simulink library "BaseOperationLib_Browser"  (Simulink 7.5)
settings: Solver=ode45  StartTime=0.0  StopTime=10.0  RelTol=1e-3
undefined symbols (not defined in the file or in its folder): DiscIntNeverNeededParam
libraries: BaseOperationLib_Browser x6, simulink x2
settings Model: Creator=zhangliming  LastModifiedBy=xinming

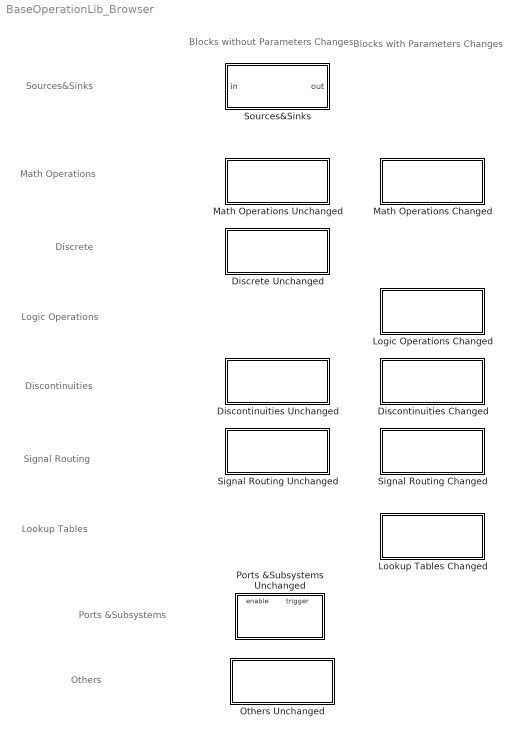
== system BaseOperationLib_Browser ==
  note: Sources&Sinks
  note: Math Operations
  note: Discrete
  note: Discontinuities
  note: Signal Routing
  note: Lookup Tables
  note: Others
  note: Ports &Subsystems
  note: Blocks without
      | Parameters Changes
  note: Blocks with
      | Parameters Changes
  note: Logic Operations
  Discontinuities Changed : Subsystem
  Discontinuities Unchanged : Subsystem
  "Discrete Unchanged " : Subsystem
  Logic Operations Changed : Subsystem
  Lookup Tables Changed : Subsystem
  Math Operations Changed : Subsystem
  Math Operations Unchanged : Subsystem
  Others Unchanged : Subsystem
  Ports &Subsystems Unchanged : Subsystem  TreatAsAtomicUnit=on
  Signal Routing Changed : Subsystem
  Signal Routing Unchanged : Subsystem
  Sources&Sinks : Subsystem

== system BaseOperationLib_Browser/Discontinuities Changed ==
  Relay : Relay  OnSwitchValue=1  OffSwitchValue=1  OutDataType=fixdt(1, 16)  OutScaling=2^0  OutDataTypeStr=Inherit: Inherit via back propagation
      settings: AttributesFormatString=%<OnSwitchValue> OnOut %<OnOutputValue>\n%<OffSwitchValue> OffOut %<OffOutputValue>
      mask Display: patch([0 1 1 1 .75], [1 1 0 .75 1], [0 1 0]);

== system BaseOperationLib_Browser/Discontinuities Unchanged ==
  RampLim : Subsystem
  Rate Limiter Dynamic : Subsystem
      mask Type: Rate Limiter Dynamic
      mask Description: Limit rising and falling rates of the signals at the second input by using the first input (upper limit) and the third input (lower limit).
      mask Display:
      | patch([0 1 1 1 .75], [1 1 0 .75 1], [0 1 0]);
      | plot([0.15 0.95],[.5 .5],[.5 .5],[0.05 0.95],0.05+0.9*[.2 .8],0.05+0.9*[0 1]);
  Saturation : Saturate  OutDataType=fixdt(1, 16)  OutScaling=2^0
      settings: AttributesFormatString=ULim:%<UpperLimit>\nLLim:%<LowerLimit>
      mask Display: patch([0 1 1 1 .75], [1 1 0 .75 1], [0 1 0]);
  Saturation Dynamic : Subsystem  mask(Saturation Dynamic){OutMin=[], OutMax=[], OutDataTypeStr=Inherit: Same as second input, OutputDataTypeScalingMode=Same as second input, OutDataType=fixdt(1, 16), OutScaling=2^-10, LockScale=off, RndMeth=Floor, DoSatur=on}
      mask prompts: OutMin "Output minimum:"; OutMax "Output maximum:"; OutDataTypeStr "Output data type:"; OutputDataTypeScalingMode "Output data type mode:"; OutDataType "Output data type (e.g. fixdt(1, 16), fixdt('single')):"; OutScaling "Output scaling (Slope, e.g. 2^-9 or [Slope Bias], e.g. [1.25 3]):"; LockScale "Lock output data type setting against changes by the fixed-point tools"; RndMeth "Integer rounding mode:"; DoSatur "Saturate on integer overflow"
      mask help: Bound the range of the second input by using the first input (upper limit) and the third input (lower limit).
      mask init:
      | blkH = gcbh;
      | blkName = getfullname(blkH);
      | 
      | switch_blks = {'Switch','Switch2'}; 
      | for i = 1:length(switch_blks)
      |   set_param([blkName,'/',switch_blks{i}], ...
      |       'RndMeth', RndMeth, ...
      | 	  'DoSatur', DoSatur);
      | end
      | 
      | propBlk = [blkName, '/Data Type Propagation'];
      | 
      | if strcmp(OutputDataTypeScalingMode, 'Same as second input')
      |     set_param(propBlk, 'PropDataTypeMode', 'Inherit via propagation rule', ...
      |                        'PropScalingMode',  'Inherit via propagation rule');
      | else
      |     scaling = OutScaling;
      |     switch OutputDataTypeScalingMode
      |       case 'double'
      |         dataType = 'fixdt(''double'')';
      |       case 'single'
      |         dataType = 'fixdt(''single'')';
      |       case 'int8'
      |         dataType = 'fixdt(1,8,0)';
      |       case 'uint8'
      |         dataType = 'fixdt(0,8,0)';
      |       case 'int16'
      |         dataType = 'fixdt(1,16,0)';
      |       case 'uint16'
      |         dataType = 'fixdt(0,16,0)';
      |       case 'int32'
      |         dataType = 'fixdt(1,32,0)';
      |       case 'uint32'
      |         dataType = 'fixdt(0,32,0)';
      |       case 'Specify via dialog'
      |         dataType = OutDataType;
      |     end
      |     
      |     set_param(propBlk, 'PropDataTypeMode', 'Specify via dialog', ...
      |                        'PropScalingMode',  'Specify via dialog', ...
      |                        'PropDataType',     dataType, ...
      |                        'PropScaling',      scaling);
      | end
      mask StyleString: min,max,unidt({m=3|4|5||6|1|2|}{i=Inherit: Same as second input}{b=double|single|int8|uint8|int16|uint16|int32|uint32}{s=UDTBinaryPointMode|UDTSlopeBiasMode}{g=UDTSignedSign|UDTUnsignedSign}),popup(double|single|int8|uint8|int16|uint16|int32|uint32|Specify via dialog|Same as second input),edit,edit,checkbox,popup(Ceiling|Convergent|Floor|Nearest|Round|Simplest|Zero),checkbox
      mask CallbackString: ||fixptdialog(gcbh)|fixptdialog(gcbh)|fixptdialog(gcbh)||||
      mask TabNameString: Signal Attributes,Signal Attributes,Signal Attributes,Signal Attributes,Signal Attributes,Signal Attributes,Signal Attributes,Signal Attributes,Signal Attributes
      mask Display:
      | patch([0 1 1 1 .75], [1 1 0 .75 1], [0 1 0]);
      | plot([0.15 0.85],[.5 .5],[.5 .5],[0.05 0.95],0.15+0.7*[0 .25 .75 1],0.05+0.9*[.25 .25 .75 .75]);
  WerghtingFilter : Subsystem

== system BaseOperationLib_Browser/Discrete Unchanged  ==
  note: Nothing else, only "limit out" could not be chose. It can be limit outside this block.
  Discrete-Time Integrator1 : DiscreteIntegrator  ExternalReset=falling  SampleTime=-1  OutDataType=PDT_s  OutDataTypeStr=Inherit: Inherit via back propagation  UpperSaturationLimit=100  LowerSaturationLimit=0  ICPrevOutput=DiscIntNeverNeededParam  ICPrevScaledInput=DiscIntNeverNeededParam
  Unit Delay : UnitDelay  SampleTime=-1
      mask Display: patch([0 1 1 1 .75], [1 1 0 .75 1], [0 1 0]);
  Unit Delay External IC : Subsystem  mask(Unit Delay External Initial Condition){tsamp=-1}
      mask prompts: tsamp "Sample time:"
      mask help:
      | Normally, the output is the signal u delayed by one sample period.
      | The initial condition is given by the signal IC.
      mask Display:
      | patch([0 1 1 1 .75], [1 1 0 .75 1], [0 1 0]);
      | dpoly(1,[1 0],'z')

== system BaseOperationLib_Browser/Logic Operations Changed ==
  Compare To Constant : Subsystem  mask(Compare To Constant){relop=<=, const=3.0, ZeroCross=on}
      mask prompts: relop "Operator:"; const "Constant value:"; ZeroCross "Enable zero-crossing detection"
      mask help: Determine how a signal compares to a constant.
      mask init:
      | blkName = gcb;
      | 
      | set_param([blkName,'/Compare'],'relop',relop, ...
      | 	 'ZeroCross', ZeroCross);
      | 
      | str = [relop,' C']; %default
      | 
      | const_str = get_param(blkName, 'const');
      | 
      | if isempty(strfind(const_str, ' ')) && isempty(strfind(const_str, ','))
      |     % scalar or single expression
      |     if isempty(str2num(const_str))
      |         %expression
      |         str = [relop, ' ', const_str];
      |     elseif length(const) == 1
      |         str = [relop,' ',num2str(double(const))];
      |     end
      | end
      mask StyleString: popup(==|~=|<|<=|>=|>),edit,checkbox
      mask CallbackString: ||sl('zeroCrossEnable', gcbh);
      mask Display:
      | patch([0 1 1 1 .75], [1 1 0 .75 1], [0 1 0]);
      | disp(str)
  Interval Test Dynamic : Subsystem  mask(Interval Test Dynamic){IntervalClosedRight=on, IntervalClosedLeft=on}
      mask prompts: IntervalClosedRight "Interval closed on right"; IntervalClosedLeft "Interval closed on left"
      mask help: If the input is in the interval between the lower limit and the upper limit, then the output is TRUE, otherwise it is FALSE.
      mask init:
      | if IntervalClosedLeft
      |   lOff = 0;
      |   lRelop = '<=';
      | else
      |   lOff = 0.1;
      |   lRelop = '<';
      | end
      | if IntervalClosedRight
      |   rOff = 0;
      |   uRelop = '<=';
      | else
      |   rOff = 0.1;
      |   uRelop = '<';
      | end
      | blkH = gcbh;
      | blkName = getfullname(gcbh);
      | 
      | set_param([blkName,'/Upper Test'],'relop',uRelop);
      | set_param([blkName,'/Lower Test'],'relop',lRelop);
      mask Display:
      | patch([0 1 1 1 .75], [1 1 0 .75 1], [0 1 0]);
      | plot(0.35+0.65*[0 1],[0.3 0.3],0.35+0.65*[0.3 0.3],[0 1],0.35+0.65*[0 0.2 0.2],[0.35 0.35 0.55-lOff],0.35+0.65*[0.2 0.2 0.55 0.55],[0.55+lOff 0.75 0.75 0.55+rOff],0.35+0.65*[0.55 0.55 1],[0.55-rOff 0.35 0.35]);
  Logical Operator : Logic  OutDataTypeMode=Specify via dialog  LogicDataType=PDT_Bool  OutDataTypeStr=PDT_Bool
      mask Display: patch([0 1 1 1 .75], [1 1 0 .75 1], [0 1 0]);
  Relational Operator : RelationalOperator  Operator=<=  LogicOutDataTypeMode=Specify via dialog  LogicDataType=PDT_Bool  OutDataTypeStr=PDT_Bool  InputSameDT=on
      mask Display: patch([0 1 1 1 .75], [1 1 0 .75 1], [0 1 0]);

== system BaseOperationLib_Browser/Lookup Tables Changed ==
  Lookup Table : Lookup  InputValues=[-5:5]  Table=tanh([-5:5])  LookUpMeth=Interpolation-Use End Values  OutDataType=fixdt(1, 16)  OutScaling=2^0  OutDataTypeStr=Inherit: Inherit via back propagation  SaturateOnIntegerOverflow=on
      settings: AttributesFormatString=X:%<InputValues>\nTAB:%<Table>
      mask Display: patch([0 1 1 1 .75], [1 1 0 .75 1], [0 1 0]);
  LookupTable (2-D) : Lookup2D  RowIndex=[1:3]  ColumnIndex=[1:3]  Table=[4 5 6;16 19 20;10 18 23]  LookUpMeth=Interpolation-Use End Values  OutDataType=fixdt(1, 16)  OutScaling=2^0  OutDataTypeStr=Inherit: Inherit via back propagation  SaturateOnIntegerOverflow=on
      settings: AttributesFormatString=X:%<RowIndex>\nY:%<ColumnIndex>\nTAB:%<Table>
      mask Display: patch([0 1 1 1 .75], [1 1 0 .75 1], [0 1 0]);

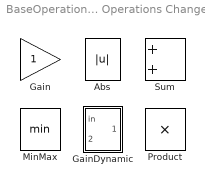
== system BaseOperationLib_Browser/Math Operations Changed ==
  Abs : Abs  OutDataType=fixdt(1, 16)  OutScaling=2^0  SaturateOnIntegerOverflow=on
      mask Display: patch([0 1 1 1 .75], [1 1 0 .75 1], [0 1 0]);
  Gain : Gain  ParameterDataType=fixdt(1, 16)  ParameterScaling=2^0  ParamDataTypeStr=Inherit: Inherit from 'Gain'  OutDataType=fixdt(1, 16)  OutScaling=2^0  SaturateOnIntegerOverflow=on  OutDataTypeStr=Inherit: Same as input
      mask Display: patch([0 1 1 1 .75], [1 1 0 .75 1], [0 1 0]);
  GainDynamic : Subsystem
      mask Type: Ratio product
      mask Description: This block is used to product a Signal with a Ratio
      mask Display:
      | patch([0 1 1 1 .75], [1 1 0 .75 1], [0 1 0]);
      | port_label('input',1,'in')
      | port_label('input',2,'ratio')
      | port_label('output',1,'out')
  MinMax : MinMax  Inputs=2  OutDataType=fixdt(1, 16)  OutScaling=2^0  SaturateOnIntegerOverflow=on  InputSameDT=on
      mask Display: patch([0 1 1 1 .75], [1 1 0 .75 1], [0 1 0]);
  Product : Product  OutDataTypeStr=Inherit: Inherit via back propagation  SaturateOnIntegerOverflow=on  RndMeth=Zero
      mask Display: patch([0 1 1 1 .75], [1 1 0 .75 1], [0 1 0]);
  Sum : Sum  OutDataType=fixdt(1, 16)  OutScaling=2^0  SaturateOnIntegerOverflow=on  InputSameDT=on  OutDataTypeStr=Inherit: Same as first input
      mask Display: patch([0 1 1 1 .75], [1 1 0 .75 1], [0 1 0]);

== system BaseOperationLib_Browser/Math Operations Unchanged ==
  Sign : Signum
      mask Display: patch([0 1 1 1 .75], [1 1 0 .75 1], [0 1 0]);

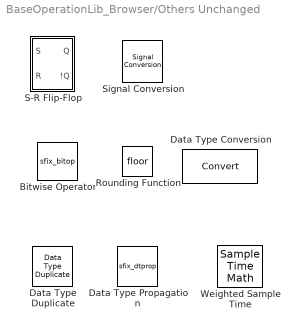
== system BaseOperationLib_Browser/Others Unchanged ==
  Bitwise Operator : S-Function  FunctionName=sfix_bitop  Parameters=UseBitMask,NumInputPorts,BitMask,BitMaskRealWorld,logicop  EnableBusSupport=off  mask(Bitwise Operator){logicop=AND, UseBitMask=on, NumInputPorts=1, BitMask=bin2dec('11011001'), BitMaskRealWorld=Stored Integer}
      mask prompts: logicop "Operator:"; UseBitMask "Use bit mask ..."; NumInputPorts "Number of input ports:"; BitMask "Bit Mask"; BitMaskRealWorld "Treat mask as:"
      mask help: Perform the specified bitwise operation on the inputs. The output data type should represent zero exactly.
      mask init:
      | str = '';
      | if UseBitMask
      |   [m,n] = size(BitMask);
      |   if ischar(BitMask)
      |     len = m;
      |     n = 1;
      |   else
      |     len = m * n;
      |   end
      |   internalBitMask = zeros(m,n);
      |   if isnumeric(BitMask)
      |     for i=1:len,
      |       internalBitMask(i) = BitMask(i);
      |     end
      |   elseif ischar(BitMask)
      |     for i=1:m,
      |       internalBitMask(i) = hex2dec(BitMask(i,:));
      |     end
      |   elseif iscell(BitMask)
      |     for i=1:len,
      |       if isnumeric( BitMask{i} )
      |         internalBitMask(i) = BitMask{i};
      |       elseif ischar( BitMask{i} )
      |         internalBitMask(i) = hex2dec(BitMask{i});
      |       else
      |         errordlg(['Data type is not supported at cell item ', num2str(i) ]);
      |       end
      |     end
      |   end
      |   BitMask = internalBitMask;
      |   for i=1:len
      |     if BitMask(i) > (2^52)-1
      |       error(DAStudio.message('Simulink:blocks:BitMaskWordLengthTooLarge')); 
      |     end
      |   end 
      |   if len == 1
      |      if BitMaskRealWorld == 1 || BitMask(1) < 0
      |        str=num2str(BitMask(1));
      |      else
      |        str=['0x',dec2hex(floor(BitMask(1)))];
      |      end
      |   else
      |      str='Masks';
      |   end
      | else
      |   BitMask = 0;
      |   str='';
      | end
      mask StyleString: popup(AND|OR|NAND|NOR|XOR|NOT),checkbox,edit,edit,popup(Real World Value|Stored Integer)
      mask CallbackString: fixptdialog(gcbh)|fixptdialog(gcbh)|||
      mask Display: fprintf(['Bitwise\n',logicop,'\n',str])
  Data Type Duplicate : DataTypeDuplicate
  Data Type Propagation : S-Function  FunctionName=sfix_dtprop  Parameters=14,PropDataTypeMode,(getdatatypespecs(PropDataType,PropScaling,DblOver,0, 0, PropDataTypeMode, PropScalingMode)),IfRefDouble,IfRefSingle,IsSigned,NumBitsBase,NumBitsMult,NumBitsAdd,(sort(reshape(round(NumBitsAllowFinal), prod(size(NumBitsAllowFinal)),1))),PropScalingMode,ValuesUsedBestPrec,SlopeBase,SlopeMult,SlopeAdd,BiasBase,BiasMult,BiasAdd,DblOver  EnableBusSupport=off  mask(Data Type Propagation){PropDataTypeMode=Inherit via propagation rule, PropDataType=fixdt(1, 16), IfRefDouble=double, IfRefSingle=single, IsSigned=IsSigned1 or IsSigned2, NumBitsBase=max([NumBits1 NumBits2]), NumBitsMult=1, NumBitsAdd=0, NumBitsAllowFinal=1:128, PropScalingMode=Inherit via propagation rule, PropScaling=2^-10, ValuesUsedBestPrec=[5 -7], SlopeBase=min([Slope1 Slope2]), SlopeMult=1, SlopeAdd=0, BiasBase=Bias1, BiasMult=1, BiasAdd=0}
      mask prompts: PropDataTypeMode "1. Propagated data type:"; PropDataType "1.1. Propagated data type (e.g. fixdt(1, 16), fixdt('single')):"; IfRefDouble "1.1. If any reference input is double, output is:"; IfRefSingle "1.2. If any reference input is single, output is:"; IsSigned "1.3. Is-Signed:"; NumBitsBase "1.4.1. Number-of-Bits: Base"; NumBitsMult "1.4.2. Number-of-Bits: Multiplicative adjustment"; NumBitsAdd "1.4.3. Number-of-Bits: Additive adjustment"; NumBitsAllowFinal "1.4.4. Number-of-Bits: Allowable final values"; PropScalingMode "2. Propagated scaling:"; PropScaling "2.1. Propagated scaling (Slope, e.g. 2^-9 or [Slope Bias], e.g. [1.25 3]):"; ValuesUsedBestPrec "2.1. Values used to determine best precision scaling."; SlopeBase "2.1.1. Slope: Base"; SlopeMult "2.1.2. Slope: Multiplicative adjustment"; SlopeAdd "2.1.3. Slope: Additive adjustment"; BiasBase "2.2.1. Bias: Base"; BiasMult "2.2.2. Bias: Multiplicative adjustment:"; BiasAdd "2.2.3. Bias: Additive adjustment:"
      mask help:
      | Set the Data Type and Scaling of the propagated signal based on information from the reference signals.
      | Notes:
      | 1) Items closer to the top of the dialog have higher priority/precedence.
      | a) Reference inputs of type double have priority over all others.
      | b) Singles have priority over integer and fixed point data types.
      | c) Multiplicative adjustments are carried out before additive adjustments.
      | d) Number-of-Bits is determined before the precision or positive-range is inherited from the reference signals.
      | 2) PosRange is one bit higher than the exact maximum positive range of the signal.
      | 3) The computed Number-of-Bits is promoted to the smallest allowable value that is greater than or equal.  If none exists, then error.
      mask init:
      | DblOver = 0;
      mask StyleString: popup(Specify via dialog|Inherit via propagation rule),edit,popup(double|single),popup(double|single),popup(IsSigned1|IsSigned2|IsSigned1 or IsSigned2|TRUE|FALSE),popup(NumBits1|NumBits2|max([NumBits1 NumBits2])|min([NumBits1 NumBits2])|NumBits1+NumBits2),edit,edit,edit,popup(Specify via dialog|Inherit via propagation rule|Obtain via best precision),edit,edit,popup(Slope1|Slope2|max([Slope1 Slope2])|min([Slope1 Slope2])|Slope1*Slope2|Slope1/Slope2|PosRange1|PosRange2|max([PosRange1 PosRange2])|min([PosRange1 PosRange2])|PosRange1*PosRange2|PosRange1/PosRange2),edit,edit,popup(Bias1|Bias2|max([Bias1 Bias2])|min([Bias1 Bias2])|Bias1*Bias2|Bias1/Bias2|Bias1+Bias2|Bias1-Bias2),edit,edit
      mask CallbackString: fixptdialog(gcbh)|fixptdialog(gcbh)||||||||fixptdialog(gcbh)||||||||
      mask TabNameString: Propagated type,Propagated type,Propagated type,Propagated type,Propagated type,Propagated type,Propagated type,Propagated type,Propagated type,Propagated scaling,Propagated scaling,Propagated scaling,Propagated scaling,Propagated scaling,Propagated scaling,Propagated scaling,Propagated scaling,Propagated scaling
      mask Display:
      | port_label('Input',1,'Ref1');
      | port_label('Input',2,'Ref2');
      | port_label('Input',3,'Prop');
  Data Type Conversion : DataTypeConversion  OutDataType=fixdt(1, 16)  OutScaling=2^0
  Rounding Function : Rounding
  S-R Flip-Flop : Subsystem  mask(SRFlipFlop){initial_condition=0}
      mask prompts: initial_condition "Initial condition (state of Q):"
      mask help: S-R Flip-Flop Block
      mask Help: web([docroot '/toolbox/simulink/ref_extras/srflipflop.html'])
      mask Display: patch([0 1 1 1 .75], [1 1 0 .75 1], [0 1 0]);
  Signal Conversion : SignalConversion  ConversionOutput=Contiguous copy
      mask Display: patch([0 1 1 1 .75], [1 1 0 .75 1], [0 1 0]);
  Weighted Sample Time : SampleTimeMath  TsampMathOp=Ts Only

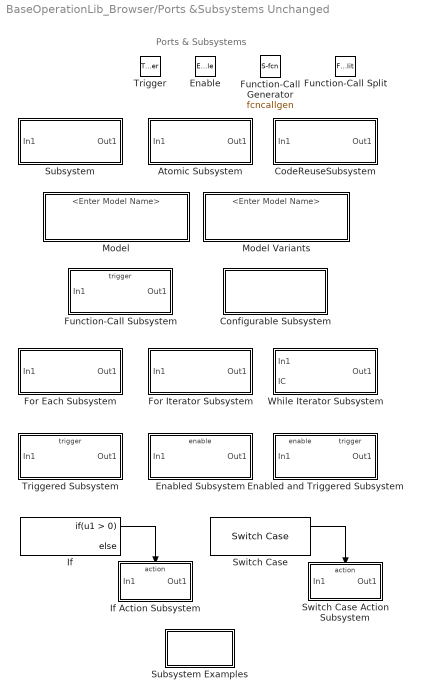
== system BaseOperationLib_Browser/Ports &Subsystems Unchanged ==
  note: Ports & Subsystems
  Enable : EnablePort
  Trigger : TriggerPort  TriggerType=falling
  Atomic Subsystem : Subsystem  TreatAsAtomicUnit=on
      settings: CopyFcn=set_param(gcbh,'LinkStatus','none'); set_param(gcbh,'Mask','off'); set_param(gcbh,'MaskType',''); set_param(gcbh,'MaskDescription',''); set_param(gcbh,'OpenFcn',''); set_param(gcbh,'CopyFcn','')  OpenFcn=open_system(gcbh,'force')
      mask Type: Atomic Subsystem
      mask Description: A subsystem block template containing an inport and outport block.
  CodeReuseSubsystem : Subsystem  TreatAsAtomicUnit=on
      settings: CopyFcn=set_param(gcbh,'LinkStatus','none'); set_param(gcbh,'Mask','off'); set_param(gcbh,'MaskType',''); set_param(gcbh,'MaskDescription',''); set_param(gcbh,'OpenFcn',''); set_param(gcbh,'CopyFcn','')  OpenFcn=open_system(gcb,'force')  RTWFcnNameOpts=Use subsystem name  RTWFileNameOpts=Use function name
      mask Type: Code Reuse Subsystem
      mask Description: A subsystem block template containing an inport and outport block.
  Configurable Subsystem : Subsystem
      settings: TemplateBlock=master
  Enabled Subsystem : Subsystem  TreatAsAtomicUnit=on
      settings: CopyFcn=set_param(gcbh,'LinkStatus','none'); set_param(gcbh,'Mask','off'); set_param(gcbh,'MaskType',''); set_param(gcbh,'MaskDescription',''); set_param(gcbh,'OpenFcn',''); set_param(gcbh,'CopyFcn','')  OpenFcn=open_system(gcbh,'force')
      mask Type: Enabled Subsystem
      mask Description: A subsystem block template containing an enable port, inport and outport block.
  Enabled and Triggered Subsystem : Subsystem  TreatAsAtomicUnit=on
      settings: CopyFcn=set_param(gcbh,'LinkStatus','none'); set_param(gcbh,'Mask','off'); set_param(gcbh,'MaskType',''); set_param(gcbh,'MaskDescription',''); set_param(gcbh,'OpenFcn',''); set_param(gcbh,'CopyFcn','')  OpenFcn=open_system(gcbh,'force')
      mask Type: Enabled And Triggered Subsystem
      mask Description: A subsystem block template containing an enable port, trigger port, inport and outport block.
  For Each Subsystem : Subsystem  TreatAsAtomicUnit=on
      settings: CopyFcn=set_param(gcbh,'LinkStatus','none'); set_param(gcbh,'Mask','off'); set_param(gcbh,'MaskType',''); set_param(gcbh,'MaskDescription',''); set_param(gcbh,'OpenFcn',''); set_param(gcbh,'CopyFcn','')  OpenFcn=open_system(gcbh,'force')
      mask Type: For Each Subsystem
      mask Description: A subsystem block template containing a for each, inport and outport block.
  For Iterator Subsystem : Subsystem  TreatAsAtomicUnit=on
      settings: CopyFcn=set_param(gcbh,'LinkStatus','none'); set_param(gcbh,'Mask','off'); set_param(gcbh,'MaskType',''); set_param(gcbh,'MaskDescription',''); set_param(gcbh,'OpenFcn',''); set_param(gcbh,'CopyFcn','')  OpenFcn=open_system(gcbh,'force')
      mask Type: For Iterator Subsystem
      mask Description: A subsystem block template containing a for iterator, inport and outport block.
  Function-Call Generator : S-Function  FunctionName=fcncallgen  Parameters=sample_time,numberOfIterations  EnableBusSupport=off  mask(Function-Call Generator){sample_time=1, numberOfIterations=1}
      mask prompts: sample_time "Sample time:"; numberOfIterations "Number of iterations:"
      mask help:
      | This block implements an iterator operation. On each time-step as defined by the sample time field, this block will execute the function-call subsystem(s) that it drives for the specified number of iterations.
      |
      | Demux the block's output to execute multiple function-call subsystems in a prescribed order.  The system connected to first demux port is executed first, the system connected to second demux port is executed second, and so on.
      mask init:
      | if ~isempty(numberOfIterations) & length(numberOfIterations) == 1 & (numberOfIterations > 1),
      | str=sprintf('iterate I = 1:%d',numberOfIterations);
      | else, str = 'f()';
      | end;
      mask Help: This block executes a function-call subsystem at the rate specified by the sample time and a specified number of times.
      mask Display: disp(str)
  Function-Call Split : FunctionCallSplit
      settings: CopyFcn=set_param(gcbh,'ShowName','off','CopyFcn','')
  Function-Call Subsystem : Subsystem  TreatAsAtomicUnit=on
      settings: CopyFcn=set_param(gcbh,'LinkStatus','none'); set_param(gcbh,'Mask','off'); set_param(gcbh,'MaskType',''); set_param(gcbh,'MaskDescription',''); set_param(gcbh,'OpenFcn',''); set_param(gcbh,'CopyFcn','')  OpenFcn=open_system(gcbh,'force')
      mask Type: Function-Call Subsystem
      mask Description: A subsystem block template containing a function-call trigger port, inport and outport block.
  If : If
  If Action Subsystem : Subsystem  TreatAsAtomicUnit=on
      settings: CopyFcn=set_param(gcbh,'LinkStatus','none'); set_param(gcbh,'Mask','off'); set_param(gcbh,'MaskType',''); set_param(gcbh,'MaskDescription',''); set_param(gcbh,'OpenFcn',''); set_param(gcbh,'CopyFcn','')  OpenFcn=open_system(gcbh,'force')
      mask Type: If Action Subsystem
      mask Description: A subsystem block template containing an action port, inport and outport block.
  Model : ModelReference  ModelNameDialog=<Enter Model Name>  SimulationMode=Accelerator
  Model Variants : ModelReference  ModelNameDialog=<Enter Model Name>  SimulationMode=Accelerator  Variant=on
      settings: AttributesFormatString=%<ActiveVariant>
  Subsystem : Subsystem
      settings: CopyFcn=set_param(gcbh,'LinkStatus','none'); set_param(gcbh,'Mask','off'); set_param(gcbh,'MaskType',''); set_param(gcbh,'MaskDescription',''); set_param(gcbh,'OpenFcn',''); set_param(gcbh,'CopyFcn','')  OpenFcn=open_system(gcbh,'force')
      mask Type: Virtual Subsystem
      mask Description: A subsystem block template containing an inport and outport block.
  Subsystem Examples : Subsystem
      settings: OpenFcn=open_system('sl_subsys_semantics','force')
      mask Type: Subsystem Examples
      mask Description: These are examples of how to use the different types of subsystems.
      mask Display: disp('Subsystem\nExamples')
  Switch Case : SwitchCase
  Switch Case Action Subsystem : Subsystem  TreatAsAtomicUnit=on
      settings: CopyFcn=set_param(gcbh,'LinkStatus','none'); set_param(gcbh,'Mask','off'); set_param(gcbh,'MaskType',''); set_param(gcbh,'MaskDescription',''); set_param(gcbh,'OpenFcn',''); set_param(gcbh,'CopyFcn','')  OpenFcn=open_system(gcbh,'force')
      mask Type: Switch Case Action Subsystem
      mask Description: A subsystem block template containing an action port, inport and outport block.
  Triggered Subsystem : Subsystem  TreatAsAtomicUnit=on
      settings: CopyFcn=set_param(gcbh,'LinkStatus','none'); set_param(gcbh,'Mask','off'); set_param(gcbh,'MaskType',''); set_param(gcbh,'MaskDescription',''); set_param(gcbh,'OpenFcn',''); set_param(gcbh,'CopyFcn','')  OpenFcn=open_system(gcbh,'force')
      mask Type: Triggered Subsystem
      mask Description: A subsystem block template containing a trigger port, inport and outport block.
  While Iterator Subsystem : Subsystem  TreatAsAtomicUnit=on
      settings: CopyFcn=set_param(gcbh,'LinkStatus','none'); set_param(gcbh,'Mask','off'); set_param(gcbh,'MaskType',''); set_param(gcbh,'MaskDescription',''); set_param(gcbh,'OpenFcn',''); set_param(gcbh,'CopyFcn','')  OpenFcn=open_system(gcbh,'force')
      mask Type: While Iterator Subsystem
      mask Description: A subsystem block template containing a while iterator, inport and outport block.
  wires:
  Switch Case/1 -> Switch Case Action Subsystem/Action
  If/1 -> If Action Subsystem/Action

== system BaseOperationLib_Browser/Signal Routing Changed ==
  Multiport Switch : MultiPortSwitch  zeroidx=off  OutDataType=fixdt(1, 16)  OutScaling=2^0  SaturateOnIntegerOverflow=on  InputSameDT=on
      mask Display: patch([0 1 1 1 .75], [1 1 0 .75 1], [0 1 0]);
  Switch : Switch  Criteria=u2 ~= 0  Threshold=1  SaturateOnIntegerOverflow=on  InputSameDT=on
      mask Display: patch([0 1 1 1 .75], [1 1 0 .75 1], [0 1 0]);

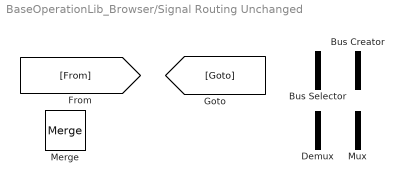
== system BaseOperationLib_Browser/Signal Routing Unchanged ==
  Bus Creator : BusCreator  Inputs=2
  Bus Selector : BusSelector  OutputSignals=signal1,signal2
  Demux : Demux  Outputs=2
  Merge : Merge
      mask Display: patch([0 1 1 1 .75], [1 1 0 .75 1], [0 1 0]);
  Mux : Mux  Inputs=2

== system BaseOperationLib_Browser/Sources&Sinks ==
  in : Inport
  Constant : Constant  Value=0  OutDataType=fixdt(1, 16)  OutScaling=2^0
      mask Display: patch([0 1 1 1 .75], [1 1 0 .75 1], [0 1 0]);
  Display : Display
  Scope : Scope
  Terminator : Terminator
  out : Outport

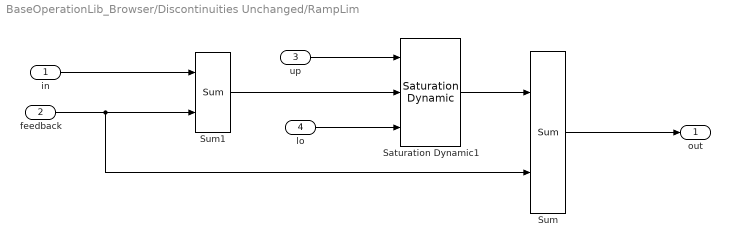
== system BaseOperationLib_Browser/Discontinuities Unchanged/RampLim ==
  in : Inport
  feedback : Inport  Port=2
  up : Inport  Port=3
  lo : Inport  Port=4
  Saturation Dynamic1 : BaseOperationLib_Browser/Discontinuities Unchanged/Saturation Dynamic  SystemSampleTime=-1  OutMin=[]  OutMax=[]  OutDataTypeStr=Inherit: Same as second input  OutDataType=fixdt(1, 16)  OutScaling=2^-10  DoSatur=off
  Sum : BaseOperationLib_Browser/Math Operations Changed/Sum  Inputs=++  InputSameDT=on  OutMin=[]  OutMax=[]  OutDataType=fixdt(1, 16)  OutScaling=2^0  SaturateOnIntegerOverflow=on
  Sum1 : BaseOperationLib_Browser/Math Operations Changed/Sum  Inputs=+-  InputSameDT=on  OutMin=[]  OutMax=[]  OutDataType=fixdt(1, 16)  OutScaling=2^0  SaturateOnIntegerOverflow=on
  out : Outport
  wires:
  lo/1 -> Saturation Dynamic1/3
  feedback/1 -> Sum1/2, Sum/2
  up/1 -> Saturation Dynamic1/1
  in/1 -> Sum1/1
  Saturation Dynamic1/1 -> Sum/1
  Sum1/1 -> Saturation Dynamic1/2
  Sum/1 -> out/1

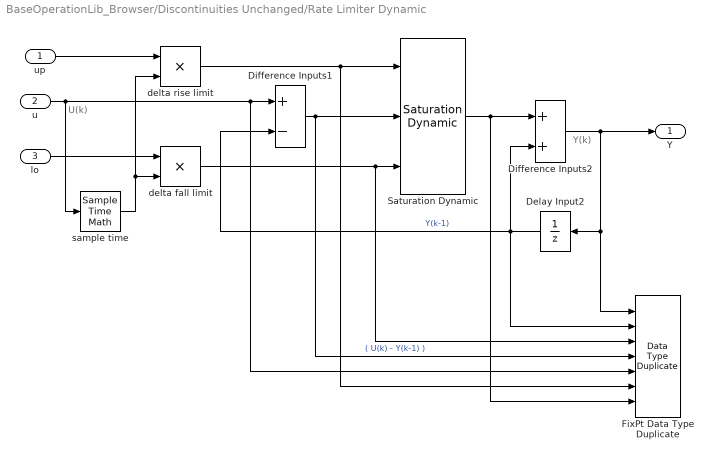
== system BaseOperationLib_Browser/Discontinuities Unchanged/Rate Limiter Dynamic ==
  note: Y(k)
  note: U(k)
  up : Inport  OutDataType=fixdt(1, 16)  OutScaling=2^0
  u : Inport  Port=2  OutDataType=fixdt(1, 16)  OutScaling=2^0
  lo : Inport  Port=3  OutDataType=fixdt(1, 16)  OutScaling=2^0
  Delay Input2 : UnitDelay  Description=Store in Global RAM  DisableCoverage=on  SampleTime=-1
  Difference Inputs1 : Sum  Description=Add in CPU  DisableCoverage=on  Inputs=+-  OutDataType=fixdt(0, 8)  OutScaling=1  OutDataTypeStr=Inherit: Inherit via back propagation
  Difference Inputs2 : Sum  Description=Add in CPU  OutDataType=fixdt(0, 8)  OutScaling=1  OutDataTypeStr=Inherit: Inherit via back propagation
  FixPt Data Type Duplicate : DataTypeDuplicate  DisableCoverage=on  NumInputPorts=7
  Saturation Dynamic : simulink/Discontinuities/Saturation Dynamic  SystemSampleTime=-1  OutMin=[]  OutMax=[]  OutDataTypeStr=Inherit: Same as second input  OutDataType=fixdt(1, 16)  OutScaling=2^-10  DoSatur=off
  delta fall limit : Product  DisableCoverage=on  Inputs=**  OutDataType=uint(16)  OutScaling=2^-10  OutDataTypeStr=Inherit: Inherit via back propagation  SaturateOnIntegerOverflow=on
  delta rise limit : Product  DisableCoverage=on  Inputs=**  OutDataType=uint(16)  OutScaling=2^-10  OutDataTypeStr=Inherit: Inherit via back propagation  SaturateOnIntegerOverflow=on
  sample time : SampleTimeMath  DisableCoverage=on  TsampMathOp=Ts Only  weightValue=1
  Y : Outport  OutDataType=fixdt(1, 16)  OutScaling=2^0  InitialOutput=0
  wires:
  Difference Inputs1/1 -> FixPt Data Type Duplicate/4, Saturation Dynamic/2  "( U(k) - Y(k-1) )"
  u/1 -> Difference Inputs1/1, FixPt Data Type Duplicate/5, sample time/1
  delta fall limit/1 -> FixPt Data Type Duplicate/3, Saturation Dynamic/3
  Saturation Dynamic/1 -> Difference Inputs2/1, FixPt Data Type Duplicate/7
  Delay Input2/1 -> Difference Inputs2/2, Difference Inputs1/2, FixPt Data Type Duplicate/2  "Y(k-1)"
  Difference Inputs2/1 -> Y/1, Delay Input2/1, FixPt Data Type Duplicate/1
  up/1 -> delta rise limit/1
  delta rise limit/1 -> FixPt Data Type Duplicate/6, Saturation Dynamic/1
  lo/1 -> delta fall limit/1
  sample time/1 -> delta fall limit/2, delta rise limit/2

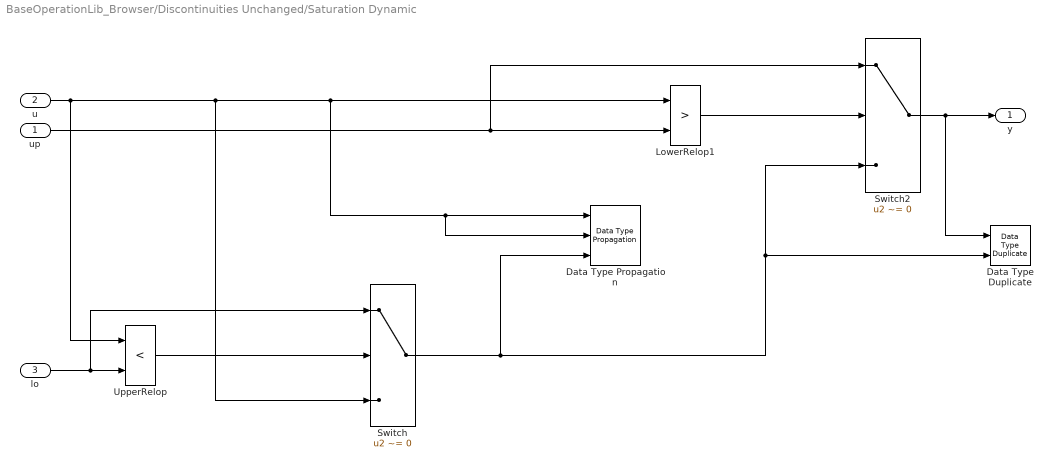
== system BaseOperationLib_Browser/Discontinuities Unchanged/Saturation Dynamic ==
  up : Inport  OutDataType=fixdt(1, 16)  OutScaling=2^0
  u : Inport  Port=2  OutDataType=fixdt(1, 16)  OutScaling=2^0
  lo : Inport  Port=3  OutDataType=fixdt(1, 16)  OutScaling=2^0
  Data Type Duplicate : DataTypeDuplicate  DisableCoverage=on
  Data Type Propagation : simulink/Signal Attributes/Data Type Propagation  PropDataType=fixdt(1, 16)  IfRefDouble=double  IfRefSingle=single  IsSigned=IsSigned1  NumBitsBase=NumBits1  NumBitsMult=1  NumBitsAdd=0  NumBitsAllowFinal=1:128  PropScaling=2^-10  ValuesUsedBestPrec=[5 -7]  SlopeBase=Slope1  SlopeMult=1  SlopeAdd=0  BiasBase=Bias1  BiasMult=1  BiasAdd=0
  LowerRelop1 : RelationalOperator  DisableCoverage=on  Operator=>  LogicOutDataTypeMode=boolean  LogicDataType=fixdt(0, 8)  OutDataTypeStr=boolean
  Switch : Switch  Criteria=u2 ~= 0  OutDataType=fixdt(1, 16)  OutScaling=2^0  OutDataTypeStr=Inherit: Inherit via back propagation  ZeroCross=off  SaturateOnIntegerOverflow=on
  Switch2 : Switch  Criteria=u2 ~= 0  OutMin=OutMin  OutMax=OutMax  OutDataType=OutDataType  OutScaling=OutScaling  OutDataTypeStr=Inherit: Inherit via back propagation  ZeroCross=off  SaturateOnIntegerOverflow=on
  UpperRelop : RelationalOperator  DisableCoverage=on  Operator=<  LogicOutDataTypeMode=boolean  LogicDataType=fixdt(0, 8)  OutDataTypeStr=boolean
  y : Outport  OutMin=OutMin  OutMax=OutMax  OutDataType=fixdt(1, 16)  OutScaling=2^0
  wires:
  up/1 -> Switch2/1, LowerRelop1/2
  u/1 -> Data Type Propagation/2, Data Type Propagation/1, LowerRelop1/1, Switch/3, UpperRelop/1
  lo/1 -> Switch/1, UpperRelop/2
  Switch/1 -> Data Type Duplicate/2, Switch2/3, Data Type Propagation/3
  Switch2/1 -> Data Type Duplicate/1, y/1
  LowerRelop1/1 -> Switch2/2
  UpperRelop/1 -> Switch/2

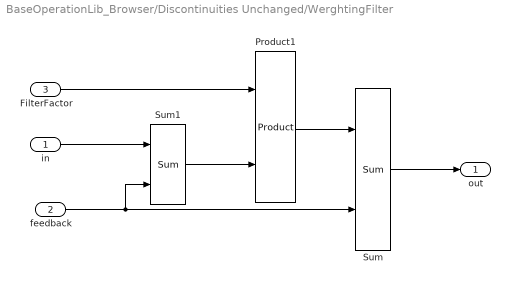
== system BaseOperationLib_Browser/Discontinuities Unchanged/WerghtingFilter ==
  in : Inport
  feedback : Inport  Port=2
  FilterFactor : Inport  Port=3
  Product1 : BaseOperationLib_Browser/Math Operations Changed/Product  Inputs=2  Multiplication=Element-wise(.*)  OutMin=[]  OutMax=[]  OutDataType=fixdt(1,16,0)  OutScaling=[]  OutDataTypeStr=Inherit: Inherit via back propagation  RndMeth=Zero  SaturateOnIntegerOverflow=on
  Sum : BaseOperationLib_Browser/Math Operations Changed/Sum  Inputs=++  InputSameDT=on  OutMin=[]  OutMax=[]  OutDataType=fixdt(1, 16)  OutScaling=2^0  SaturateOnIntegerOverflow=on
  Sum1 : BaseOperationLib_Browser/Math Operations Changed/Sum  Inputs=+-  InputSameDT=on  OutMin=[]  OutMax=[]  OutDataType=fixdt(1, 16)  OutScaling=2^0  SaturateOnIntegerOverflow=on
  out : Outport
  wires:
  Sum1/1 -> Product1/2
  Product1/1 -> Sum/1
  feedback/1 -> Sum/2, Sum1/2
  Sum/1 -> out/1
  in/1 -> Sum1/1
  FilterFactor/1 -> Product1/1

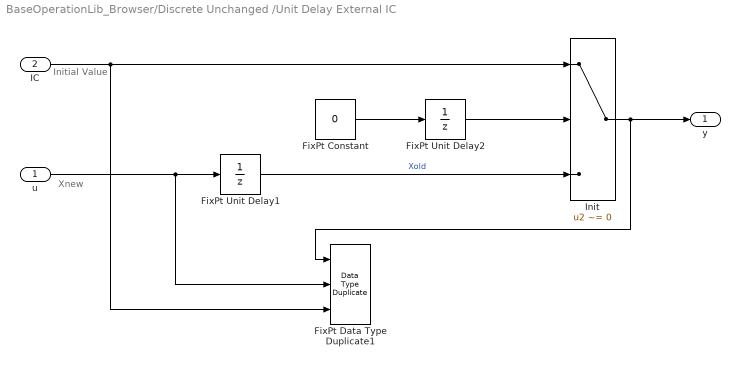
== system BaseOperationLib_Browser/Discrete Unchanged /Unit Delay External IC ==
  note: Initial Value
  note: Xnew
  u : Inport  OutDataType=fixdt(1, 16)  OutScaling=2^0
  IC : Inport  Port=2  OutDataType=fixdt(1, 16)  OutScaling=2^0
  FixPt Constant : Constant  DisableCoverage=on  Value=0  OutDataTypeMode=Specify via dialog  OutDataType=fixdt(0,8,0)  ConRadixGroup=Best Precision: Vector-wise  OutDataTypeStr=fixdt(0,8,0)
  FixPt Data Type Duplicate1 : DataTypeDuplicate  DisableCoverage=on  NumInputPorts=3
  FixPt Unit Delay1 : UnitDelay  DisableCoverage=on  X0=0.0  SampleTime=tsamp
  FixPt Unit Delay2 : UnitDelay  DisableCoverage=on  X0=1  SampleTime=tsamp
  Init : Switch  Criteria=u2 ~= 0  OutDataType=fixdt(1, 16)  OutScaling=2^0  OutDataTypeStr=Inherit: Inherit via back propagation  ZeroCross=off
  y : Outport  OutDataType=fixdt(1, 16)  OutScaling=2^0
  wires:
  IC/1 -> FixPt Data Type Duplicate1/3, Init/1
  u/1 -> FixPt Data Type Duplicate1/2, FixPt Unit Delay1/1
  FixPt Constant/1 -> FixPt Unit Delay2/1
  FixPt Unit Delay2/1 -> Init/2
  Init/1 -> FixPt Data Type Duplicate1/1, y/1
  FixPt Unit Delay1/1 -> Init/3  "Xold"

== system BaseOperationLib_Browser/Logic Operations Changed/Compare To Constant ==
  u : Inport  OutDataType=fixdt(1, 16)  OutScaling=2^0
  Compare : RelationalOperator  Operator=<=  LogicOutDataTypeMode=Specify via dialog  LogicDataType=PDT_Bool  OutDataTypeStr=PDT_Bool  InputSameDT=on
  Constant : Constant  DisableCoverage=on  Value=const  OutDataType=fixdt(1, 16)  OutScaling=1  OutDataTypeStr=Inherit: Inherit via back propagation
  y : Outport  OutDataType=fixdt(1, 16)  OutScaling=2^0
  wires:
  u/1 -> Compare/1
  Constant/1 -> Compare/2
  Compare/1 -> y/1

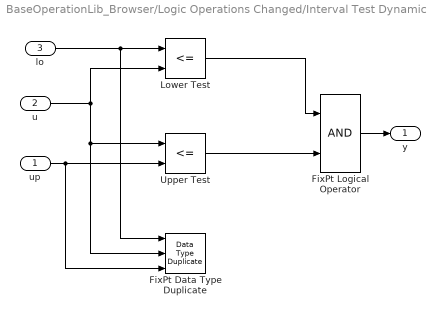
== system BaseOperationLib_Browser/Logic Operations Changed/Interval Test Dynamic ==
  up : Inport  OutDataType=fixdt(1, 16)  OutScaling=2^0
  u : Inport  Port=2  OutDataType=fixdt(1, 16)  OutScaling=2^0
  lo : Inport  Port=3  OutDataType=fixdt(1, 16)  OutScaling=2^0
  FixPt Data Type Duplicate : DataTypeDuplicate  DisableCoverage=on  NumInputPorts=3
  FixPt Logical Operator : Logic  OutDataTypeMode=Specify via dialog  LogicDataType=PDT_Bool  OutDataTypeStr=PDT_Bool
  Lower Test : RelationalOperator  DisableCoverage=on  Operator=<=  LogicOutDataTypeMode=Specify via dialog  LogicDataType=PDT_Bool  OutDataTypeStr=PDT_Bool  ZeroCross=off  InputSameDT=on
  Upper Test : RelationalOperator  DisableCoverage=on  Operator=<=  LogicOutDataTypeMode=Specify via dialog  LogicDataType=PDT_Bool  OutDataTypeStr=PDT_Bool  ZeroCross=off  InputSameDT=on
  y : Outport  OutDataType=fixdt(1, 16)  OutScaling=2^0
  wires:
  lo/1 -> FixPt Data Type Duplicate/1, Lower Test/1
  up/1 -> FixPt Data Type Duplicate/3, Upper Test/2
  Lower Test/1 -> FixPt Logical Operator/1
  Upper Test/1 -> FixPt Logical Operator/2
  u/1 -> FixPt Data Type Duplicate/2, Upper Test/1, Lower Test/2
  FixPt Logical Operator/1 -> y/1

== system BaseOperationLib_Browser/Math Operations Changed/GainDynamic ==
  in : Inport
  ratio : Inport  Port=2
  Product : Product  OutDataType=fixdt(1, 16)  OutScaling=2^0  SaturateOnIntegerOverflow=on  RndMeth=Zero  OutDataTypeStr=Inherit: Same as first input
  out : Outport
  wires:
  in/1 -> Product/1
  Product/1 -> out/1
  ratio/1 -> Product/2

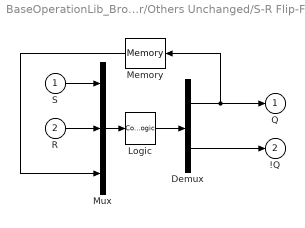
== system BaseOperationLib_Browser/Others Unchanged/S-R Flip-Flop ==
  S : Inport  OutDataType=sfix(16)  OutScaling=2^0
  R : Inport  Port=2  OutDataType=sfix(16)  OutScaling=2^0
  Demux : Demux  Outputs=2
  Logic : CombinatorialLogic  TruthTable=[0 1;1 0;0 1;0 1;1 0;1 0;0 0;0 0]
  Memory : Memory  X0=initial_condition  InheritSampleTime=on
  Mux : Mux  Inputs=3
  Q : Outport  OutDataType=sfix(16)  OutScaling=2^0  InitialOutput=0
  !Q : Outport  Port=2  OutDataType=sfix(16)  OutScaling=2^0  InitialOutput=1
  wires:
  Memory/1 -> Mux/3
  Mux/1 -> Logic/1
  Logic/1 -> Demux/1
  Demux/2 -> !Q/1
  Demux/1 -> Q/1, Memory/1
  S/1 -> Mux/1
  R/1 -> Mux/2

== system BaseOperationLib_Browser/Ports &Subsystems Unchanged/Atomic Subsystem ==
  In1 : Inport  OutDataType=fixdt(1, 16)  OutScaling=2^0
  Out1 : Outport  OutDataType=fixdt(1, 16)  OutScaling=2^0
  wires:
  In1/1 -> Out1/1

== system BaseOperationLib_Browser/Ports &Subsystems Unchanged/CodeReuseSubsystem ==
  In1 : Inport  OutDataType=fixdt(1, 16)  OutScaling=2^0
  Out1 : Outport  OutDataType=fixdt(1, 16)  OutScaling=2^0
  wires:
  In1/1 -> Out1/1

== system BaseOperationLib_Browser/Ports &Subsystems Unchanged/Configurable Subsystem ==

== system BaseOperationLib_Browser/Ports &Subsystems Unchanged/Enabled Subsystem ==
  In1 : Inport  OutDataType=fixdt(1, 16)  OutScaling=2^0
  Enable : EnablePort
  Out1 : Outport  OutDataType=fixdt(1, 16)  OutScaling=2^0
  wires:
  In1/1 -> Out1/1

== system BaseOperationLib_Browser/Ports &Subsystems Unchanged/Enabled and Triggered Subsystem ==
  In1 : Inport  OutDataType=fixdt(1, 16)  OutScaling=2^0
  Enable : EnablePort
  Trigger : TriggerPort
  Out1 : Outport  OutDataType=fixdt(1, 16)  OutScaling=2^0
  wires:
  In1/1 -> Out1/1

== system BaseOperationLib_Browser/Ports &Subsystems Unchanged/For Each Subsystem ==
  In1 : Inport  OutDataType=fixdt(1, 16)  OutScaling=2^0  Partition=on  PartitionDimension=1  PartitionWidth=1
  For Each : ForEach  DisableCoverage=on  IndexMode=One-based
  Out1 : Outport  OutDataType=fixdt(1, 16)  OutScaling=2^0  ConcatenationDimension=1
  wires:
  In1/1 -> Out1/1

== system BaseOperationLib_Browser/Ports &Subsystems Unchanged/For Iterator Subsystem ==
  In1 : Inport  OutDataType=fixdt(1, 16)  OutScaling=2^0
  For Iterator : ForIterator
  Out1 : Outport  OutDataType=fixdt(1, 16)  OutScaling=2^0
  wires:
  In1/1 -> Out1/1

== system BaseOperationLib_Browser/Ports &Subsystems Unchanged/Function-Call Subsystem ==
  In1 : Inport  OutDataType=fixdt(1, 16)  OutScaling=2^0
  function : TriggerPort  TriggerType=function-call
  Out1 : Outport  OutDataType=fixdt(1, 16)  OutScaling=2^0
  wires:
  In1/1 -> Out1/1

== system BaseOperationLib_Browser/Ports &Subsystems Unchanged/If Action Subsystem ==
  In1 : Inport  OutDataType=fixdt(1, 16)  OutScaling=2^0
  Action Port : ActionPort
  Out1 : Outport  OutDataType=fixdt(1, 16)  OutScaling=2^0
  wires:
  In1/1 -> Out1/1

== system BaseOperationLib_Browser/Ports &Subsystems Unchanged/Subsystem ==
  In1 : Inport  OutDataType=fixdt(1, 16)  OutScaling=2^0
  Out1 : Outport  OutDataType=fixdt(1, 16)  OutScaling=2^0
  wires:
  In1/1 -> Out1/1

== system BaseOperationLib_Browser/Ports &Subsystems Unchanged/Subsystem Examples ==
  Gain : Gain  ParameterDataType=fixdt(1, 16)  ParameterScaling=2^0  OutDataType=fixdt(1, 16)  OutScaling=2^0  SaturateOnIntegerOverflow=on  OutDataTypeStr=Inherit: Same as input  ParamDataTypeStr=Inherit: Same as input

== system BaseOperationLib_Browser/Ports &Subsystems Unchanged/Switch Case Action Subsystem ==
  In1 : Inport  OutDataType=fixdt(1, 16)  OutScaling=2^0
  Action Port : ActionPort
  Out1 : Outport  OutDataType=fixdt(1, 16)  OutScaling=2^0
  wires:
  In1/1 -> Out1/1

== system BaseOperationLib_Browser/Ports &Subsystems Unchanged/Triggered Subsystem ==
  In1 : Inport  OutDataType=fixdt(1, 16)  OutScaling=2^0
  Trigger : TriggerPort
  Out1 : Outport  OutDataType=fixdt(1, 16)  OutScaling=2^0
  wires:
  In1/1 -> Out1/1

== system BaseOperationLib_Browser/Ports &Subsystems Unchanged/While Iterator Subsystem ==
  In1 : Inport  OutDataType=fixdt(1, 16)  OutScaling=2^0
  IC : Inport  Port=2  OutDataType=fixdt(1, 16)  OutScaling=2^0
  While Iterator : WhileIterator
  Out1 : Outport  OutDataType=fixdt(1, 16)  OutScaling=2^0
  wires:
  IC/1 -> While Iterator/2
  In1/1 -> Out1/1
